simulink model "Likitha_Version_3_1"  (R2025b)
settings: Solver=VariableStepAuto  StartTime=0.0  StopTime=0.3  RelTol=1e-3
undefined symbols (not defined in the file): Ion, Lithium
libraries: spsBatteryLib x50, spsSeriesRLCBranchLib x15, spsCurrentMeasurementLib x10, spsVoltageMeasurementLib x10, spsIdealSwitchLib x9, spsMosfetLib x7, slpidlib x4, spsPWMGeneratorDCDCLib x2, spspowerguiLib x2, spsACVoltageSourceLib x1, eeHysteresisControl x1, spsDCMachineLib x1
(part 2 of 3)

== system Likitha_Version_3_1/Subsystem/Pulse Generator ==
  N,ref : Inport
  N,actual : Inport  Port=2
  Discrete PID Controller : slpidlib/PID Controller  Controller=PI  Form=Parallel  TimeDomain=Discrete-time  UseExternalTs=off  SampleTime=-1  IntegratorMethod=Forward Euler  FilterMethod=Forward Euler  ControllerParametersSource=internal  P=0.002  I=3e-3  UseKiTs=off  D=0  UseExternalDerivativeSource=off  N=100  UseFilter=on  TunerSelectOption=Transfer Function Based (PID Tuner App)  InitialConditionSource=internal  InitialConditionForIntegrator=0  InitialConditionForFilter=0  DifferentiatorICPrevScaledInput=0  ExternalReset=none  TrackingMode=off  Kt=1  LimitOutput=off  SatLimitsSource=internal  UpperSaturationLimit=inf  LowerSaturationLimit=-inf  LinearizeAsGain=off  AntiWindupMode=none  Kb=1  LimitIntegrator=off  UpperIntegratorSaturationLimit=inf  LowerIntegratorSaturationLimit=-inf  POutMin=[]  POutMax=[]  IOutMin=[]  IOutMax=[]  DOutMin=[]  DOutMax=[]  NOutMin=[]  NOutMax=[]  SumOutMin=[]  SumOutMax=[]  SaturationOutMin=[]  SaturationOutMax=[]  PParamMin=[]  PParamMax=[]  IParamMin=[]  IParamMax=[]  DParamMin=[]  DParamMax=[]  NParamMin=[]  NParamMax=[]  KbParamMin=[]  KbParamMax=[]  KtParamMin=[]  KtParamMax=[]  KbOutMin=[]  KbOutMax=[]  KtOutMin=[]  KtOutMax=[]  IntegratorOutMin=[]  IntegratorOutMax=[]  FilterOutMin=[]  FilterOutMax=[]  SumI1OutMin=[]  SumI1OutMax=[]  SumI2OutMin=[]  SumI2OutMax=[]  SumI3OutMin=[]  SumI3OutMax=[]  SumI4OutMin=[]  SumI4OutMax=[]  SumDOutMin=[]  SumDOutMax=[]  DifferentiatorOutMin=[]  DifferentiatorOutMax=[]  FilterDiffOutCoefMin=[]  FilterDiffOutCoefMax=[]  ReciprocalOutMin=[]  ReciprocalOutMax=[]  SumDenOutMin=[]  SumDenOutMax=[]  SumNumOutMin=[]  SumNumOutMax=[]  DivideOutMin=[]  DivideOutMax=[]  UdiffTsProdOutMin=[]  UdiffTsProdOutMax=[]  NTsProdOutMin=[]  NTsProdOutMax=[]  UintegralTsProdOutMin=[]  UintegralTsProdOutMax=[]  UngainTsProdOutMin=[]  UngainTsProdOutMax=[]  ClampingZeroOutDataTypeStr=Inherit: Inherit via back propagation  ClampingZeroOutMin=[]  ClampingZeroOutMax=[]  FilterDenConstantOutDataTypeStr=Inherit: Inherit via back propagation  FilterDenConstantOutMin=[]  FilterDenConstantOutMax=[]  PCopyOutDataTypeStr=Inherit: Inherit via back propagation  PCopyOutMin=[]  PCopyOutMax=[]  NCopyOutDataTypeStr=Inherit: Inherit via back propagation  NCopyOutMin=[]  NCopyOutMax=[]  IntegratorContinuousStateAttributes=''  IntegratorStateMustResolveToSignalObject=off  IntegratorRTWStateStorageClass=Auto  FilterContinuousStateAttributes=''  FilterStateMustResolveToSignalObject=off  FilterRTWStateStorageClass=Auto  ParallelPVariant=InternalParameters  IdealPVariant=Disabled  IVariant=InternalParameters  DVariant=Disabled  IntegratorVariant=Discrete  SatVariant=Disabled  AWVariant=Passthrough  PCopyVariant=Disabled  TRVariant=Disabled  FdbkBlocksVariant=Forward  IdealPFdbkVariant=Disabled  SatFdbkVariant=Disabled  DerivativeFilterVariant=Disabled  NVariant=Disabled  NCopyVariant=Disabled_SignalSpec  FilterICVariant=Disabled  IntegratorICVariant=InternalICs  ExternalResetVariant=Disabled  TRSumVariant=Passthrough  SumFdbkVariant=Disabled  SumVariant=Sum_PI  TsampFilterVariant=InternalTs  TsampNgainVariant=Passthrough  TsampIntegralVariant=Disabled_SignalSpec  ExternalSaturationOutDataTypeStr=Inherit: Same as second input  DerivativeSourceVariant=Disabled  PreIntVariant=InternalPreInt
  Gain : Gain  Gain=0.9
  Relational Operator : RelationalOperator  OutDataTypeStr=boolean  RndMeth=Simplest  InputSameDT=off
  Saturation : Saturate  UpperLimit=1  LowerLimit=-1
  Sawtooth Generator : spsSawtoothGeneratorLib/Sawtooth Generator  Freq=2e3  Phase=0  Ts=0
  Subtract : Sum  Inputs=+-
  pulse : Outport
  wires:
  Gain/1 -> Relational Operator/1
  Subtract/1 -> Discrete PID Controller/1
  Sawtooth Generator/1 -> Relational Operator/2
  Discrete PID Controller/1 -> Saturation/1
  Saturation/1 -> Gain/1
  Relational Operator/1 -> pulse/1
  N,actual/1 -> Subtract/2
  N,ref/1 -> Subtract/1

== system Likitha_Version_3_1/Subsystem11/1 ==
  Battery1 : spsBatteryLib/Battery  BatType=Lithium-Ion  NomV=3.3  NomQ=2.5  SOC=60  Batt_Tr=30  PresetModel=off  MaxQ=2.5  MinV=2.475  FullV=3.8412  Dis_rate=1.1739  R=0.05  Normal_OP=2.4417  expZone="[3.5653     0.13265]"
  Bus Selector : BusSelector  OutputSignals=SOC (%),Current (A),Voltage (V)
  Product : Product
  Scope : Scope  NumInputPorts=4
      settings: ActiveDisplayYMinimum=50.396039603960396  ActiveDisplayYMaximum=70.396039603960389
  Series RLC Branch : spsSeriesRLCBranchLib/Series RLC Branch  LConnTagsString=__new0  RConnTagsString=__new0  BranchType=R  Resistance=10  Inductance=1e-3  SetiL0=off  InitialCurrent=0  Capacitance=1e-6  Setx0=off  InitialVoltage=0  Measurements=None
  powergui : spspowerguiLib/powergui  Priority=1  SimulationMode=Continuous  SampleTime=50e-6  frequency=60  Iterations=50  frequencyindice=60  Pbase=100e6  ErrMax=1e-4  UnitsV=kV  UnitsW=MW  buscounter=0  FunctionMessages=off  echomessages=off  EnableUseOfTLC=off  CurrentSourceSwitches=off  DisableSnubberDevices=off  DisableRonSwitches=off  DisableVfSwitches=off  DisplayEquations=off  AutomaticDiscreteSolvers=off  SolverType=Tustin/Backward Euler (TBE)  Interpol=off  ExternalGateDelay=off  methode=off  Ts=100  x0status=blocks  SPID=on  SwTol=0  HookPort=off  NonlinearTolerance=1e-4  nMaxIteration=100  ContinueOnMaxIteration=off  RestoreLinks=warning  ResistiveCurrentMeasurement=off  Frange=[0:2:500]  Ylog=off  Xlog=on  ShowGrid=off  save=off  variable=ZData  structure=0  ZoomFFT=off  StartTime=0.0  cycles=1  DisplayStyle=1  fundamental=60  FreqAxis=off  MaxFrequency=1000  frequencyindicesteady=1  RmsSteady=1  display=off
  + : PMIOPort  Side=Right
  - : PMIOPort  Port=2  Side=Right
  tag scope: cm_1=global, soc1=global, vm_1=global
  wires:
  Battery1/1 -> Bus Selector/1
  Bus Selector/3 -> [vm_1], Scope/3, Product/2  "<Voltage (V)>"
  Bus Selector/1 -> [soc1], Scope/1  "<SOC (%)>"
  Bus Selector/2 -> [cm_1], Scope/2, Product/1  "<Current (A)>"
  Product/1 -> Scope/4
  connections:
  -/RConn1 -- Battery1/LConn2 -- Series RLC Branch/RConn1
  +/RConn1 -- Battery1/LConn1 -- Series RLC Branch/LConn1

== system Likitha_Version_3_1/Subsystem11/10 ==
  Battery1 : spsBatteryLib/Battery  BatType=Lithium-Ion  NomV=3.3  NomQ=2.7  SOC=95.5  Batt_Tr=30  PresetModel=on  MaxQ=2.7  MinV=2.475  FullV=3.8412  Dis_rate=1.1739  R=0.012222  Normal_OP=2.4417  expZone="[3.5653     0.13265]"
  Bus Selector : BusSelector  OutputSignals=SOC (%),Current (A),Voltage (V)
  Product : Product
  Scope : Scope  NumInputPorts=4
      settings: ActiveDisplayYMinimum=99.92989  ActiveDisplayYMaximum=100.00779
  + : PMIOPort  Side=Right
  - : PMIOPort  Port=2  Side=Right
  tag scope: cm_10=global, soc10=global, vm_10=global
  wires:
  Battery1/1 -> Bus Selector/1
  Bus Selector/1 -> [soc10], Scope/1  "<SOC (%)>"
  Product/1 -> Scope/4
  Bus Selector/2 -> [cm_10], Product/1, Scope/2  "<Current (A)>"
  Bus Selector/3 -> [vm_10], Scope/3, Product/2  "<Voltage (V)>"
  connections:
  +/RConn1 -- Battery1/LConn1
  -/RConn1 -- Battery1/LConn2

== system Likitha_Version_3_1/Subsystem11/11 ==
  Battery1 : spsBatteryLib/Battery  BatType=Lithium-Ion  NomV=3.3  NomQ=2.7  SOC=90  Batt_Tr=30  PresetModel=on  MaxQ=2.7  MinV=2.475  FullV=3.8412  Dis_rate=1.1739  R=0.012222  Normal_OP=2.4417  expZone="[3.5653     0.13265]"
  Bus Selector : BusSelector  OutputSignals=SOC (%),Current (A),Voltage (V)
  Product : Product
  Scope : Scope  NumInputPorts=4
      settings: ActiveDisplayYMinimum=99.92989  ActiveDisplayYMaximum=100.00779
  Series RLC Branch : spsSeriesRLCBranchLib/Series RLC Branch  LConnTagsString=__new0  RConnTagsString=__new0  BranchType=R  Resistance=0.01  Inductance=1e-3  SetiL0=off  InitialCurrent=0  Capacitance=1e-6  Setx0=off  InitialVoltage=0  Measurements=None
  + : PMIOPort  Side=Right
  - : PMIOPort  Port=2  Side=Right
  tag scope: cm_11=global, soc11=global, vm_11=global
  wires:
  Battery1/1 -> Bus Selector/1
  Bus Selector/1 -> [soc11], Scope/1  "<SOC (%)>"
  Product/1 -> Scope/4
  Bus Selector/2 -> [cm_11], Product/1, Scope/2  "<Current (A)>"
  Bus Selector/3 -> [vm_11], Scope/3, Product/2  "<Voltage (V)>"
  connections:
  -/RConn1 -- Battery1/LConn2
  Series RLC Branch/LConn1 -- Battery1/LConn1
  Series RLC Branch/RConn1 -- +/RConn1

== system Likitha_Version_3_1/Subsystem11/12 ==
  Battery1 : spsBatteryLib/Battery  BatType=Lithium-Ion  NomV=3.264  NomQ=2.61  SOC=81  Batt_Tr=30  PresetModel=on  MaxQ=2.61  MinV=2.448  FullV=3.7993  Dis_rate=1.1348  R=0.012506  Normal_OP=2.3603  expZone="[3.5264     0.12823]"
  Bus Selector : BusSelector  OutputSignals=SOC (%),Current (A),Voltage (V)
  Product : Product
  Scope : Scope  NumInputPorts=4
      settings: ActiveDisplayYMinimum=99.92989  ActiveDisplayYMaximum=100.00779
  + : PMIOPort  Side=Right
  - : PMIOPort  Port=2  Side=Right
  tag scope: cm_20=global, soc20=global, vm_20=global
  wires:
  Battery1/1 -> Bus Selector/1
  Bus Selector/1 -> [soc20], Scope/1  "<SOC (%)>"
  Product/1 -> Scope/4
  Bus Selector/2 -> [cm_20], Product/1, Scope/2  "<Current (A)>"
  Bus Selector/3 -> [vm_20], Scope/3, Product/2  "<Voltage (V)>"
  connections:
  +/RConn1 -- Battery1/LConn1
  -/RConn1 -- Battery1/LConn2

== system Likitha_Version_3_1/Subsystem11/13 ==
  Battery1 : spsBatteryLib/Battery  BatType=Lithium-Ion  NomV=3.296  NomQ=2.69  SOC=89  Batt_Tr=30  PresetModel=on  MaxQ=2.69  MinV=2.472  FullV=3.8365  Dis_rate=1.1696  R=0.012253  Normal_OP=2.4327  expZone="[3.561     0.13216]"
  Bus Selector : BusSelector  OutputSignals=SOC (%),Current (A),Voltage (V)
  Product : Product
  Scope : Scope  NumInputPorts=4
      settings: ActiveDisplayYMinimum=99.92989  ActiveDisplayYMaximum=100.00779
  + : PMIOPort  Side=Right
  - : PMIOPort  Port=2  Side=Right
  tag scope: cm_12=global, soc12=global, vm_12=global
  wires:
  Battery1/1 -> Bus Selector/1
  Bus Selector/1 -> [soc12], Scope/1  "<SOC (%)>"
  Product/1 -> Scope/4
  Bus Selector/2 -> [cm_12], Product/1, Scope/2  "<Current (A)>"
  Bus Selector/3 -> [vm_12], Scope/3, Product/2  "<Voltage (V)>"
  connections:
  +/RConn1 -- Battery1/LConn1
  -/RConn1 -- Battery1/LConn2

== system Likitha_Version_3_1/Subsystem11/14 ==
  Battery1 : spsBatteryLib/Battery  BatType=Lithium-Ion  NomV=3.292  NomQ=2.68  SOC=88  Batt_Tr=30  PresetModel=on  MaxQ=2.68  MinV=2.469  FullV=3.8318  Dis_rate=1.1652  R=0.012284  Normal_OP=2.4237  expZone="[3.5566     0.13167]"
  Bus Selector : BusSelector  OutputSignals=SOC (%),Current (A),Voltage (V)
  Product : Product
  Scope : Scope  NumInputPorts=4
      settings: ActiveDisplayYMinimum=99.92989  ActiveDisplayYMaximum=100.00779
  + : PMIOPort  Side=Right
  - : PMIOPort  Port=2  Side=Right
  tag scope: cm_13=global, soc13=global, vm_13=global
  wires:
  Battery1/1 -> Bus Selector/1
  Bus Selector/1 -> [soc13], Scope/1  "<SOC (%)>"
  Product/1 -> Scope/4
  Bus Selector/2 -> [cm_13], Product/1, Scope/2  "<Current (A)>"
  Bus Selector/3 -> [vm_13], Scope/3, Product/2  "<Voltage (V)>"
  connections:
  +/RConn1 -- Battery1/LConn1
  -/RConn1 -- Battery1/LConn2

== system Likitha_Version_3_1/Subsystem11/15 ==
  Battery1 : spsBatteryLib/Battery  BatType=Lithium-Ion  NomV=3.288  NomQ=2.67  SOC=87  Batt_Tr=30  PresetModel=on  MaxQ=2.67  MinV=2.466  FullV=3.8272  Dis_rate=1.1609  R=0.012315  Normal_OP=2.4146  expZone="[3.5523     0.13118]"
  Bus Selector : BusSelector  OutputSignals=SOC (%),Current (A),Voltage (V)
  Product : Product
  Scope : Scope  NumInputPorts=4
      settings: ActiveDisplayYMinimum=99.92989  ActiveDisplayYMaximum=100.00779
  + : PMIOPort  Side=Right
  - : PMIOPort  Port=2  Side=Right
  tag scope: cm_14=global, soc14=global, vm_14=global
  wires:
  Battery1/1 -> Bus Selector/1
  Bus Selector/1 -> [soc14], Scope/1  "<SOC (%)>"
  Product/1 -> Scope/4
  Bus Selector/2 -> [cm_14], Product/1, Scope/2  "<Current (A)>"
  Bus Selector/3 -> [vm_14], Scope/3, Product/2  "<Voltage (V)>"
  connections:
  +/RConn1 -- Battery1/LConn1
  -/RConn1 -- Battery1/LConn2

== system Likitha_Version_3_1/Subsystem11/16 ==
  Battery1 : spsBatteryLib/Battery  BatType=Lithium-Ion  NomV=3.284  NomQ=2.66  SOC=86  Batt_Tr=30  PresetModel=on  MaxQ=2.66  MinV=2.463  FullV=3.8225  Dis_rate=1.1565  R=0.012346  Normal_OP=2.4056  expZone="[3.548     0.13069]"
  Bus Selector : BusSelector  OutputSignals=SOC (%),Current (A),Voltage (V)
  Product : Product
  Scope : Scope  NumInputPorts=4
      settings: ActiveDisplayYMinimum=99.92989  ActiveDisplayYMaximum=100.00779
  + : PMIOPort  Side=Right
  - : PMIOPort  Port=2  Side=Right
  tag scope: cm_15=global, soc15=global, vm_15=global
  wires:
  Battery1/1 -> Bus Selector/1
  Bus Selector/1 -> [soc15], Scope/1  "<SOC (%)>"
  Product/1 -> Scope/4
  Bus Selector/2 -> [cm_15], Product/1, Scope/2  "<Current (A)>"
  Bus Selector/3 -> [vm_15], Scope/3, Product/2  "<Voltage (V)>"
  connections:
  +/RConn1 -- Battery1/LConn1
  -/RConn1 -- Battery1/LConn2

== system Likitha_Version_3_1/Subsystem11/17 ==
  Battery1 : spsBatteryLib/Battery  BatType=Lithium-Ion  NomV=3.28  NomQ=2.65  SOC=85  Batt_Tr=30  PresetModel=on  MaxQ=2.65  MinV=2.46  FullV=3.8179  Dis_rate=1.1522  R=0.012377  Normal_OP=2.3965  expZone="[3.5437      0.1302]"
  Bus Selector : BusSelector  OutputSignals=SOC (%),Current (A),Voltage (V)
  Product : Product
  Scope : Scope  NumInputPorts=4
      settings: ActiveDisplayYMinimum=99.92989  ActiveDisplayYMaximum=100.00779
  + : PMIOPort  Side=Right
  - : PMIOPort  Port=2  Side=Right
  tag scope: cm_16=global, soc16=global, vm_16=global
  wires:
  Battery1/1 -> Bus Selector/1
  Bus Selector/1 -> [soc16], Scope/1  "<SOC (%)>"
  Product/1 -> Scope/4
  Bus Selector/2 -> [cm_16], Product/1, Scope/2  "<Current (A)>"
  Bus Selector/3 -> [vm_16], Scope/3, Product/2  "<Voltage (V)>"
  connections:
  +/RConn1 -- Battery1/LConn1
  -/RConn1 -- Battery1/LConn2

== system Likitha_Version_3_1/Subsystem11/18 ==
  Battery1 : spsBatteryLib/Battery  BatType=Lithium-Ion  NomV=3.276  NomQ=2.64  SOC=84  Batt_Tr=30  PresetModel=on  MaxQ=2.64  MinV=2.457  FullV=3.8132  Dis_rate=1.1478  R=0.012409  Normal_OP=2.3875  expZone="[3.5393      0.1297]"
  Bus Selector : BusSelector  OutputSignals=SOC (%),Current (A),Voltage (V)
  Product : Product
  Scope : Scope  NumInputPorts=4
      settings: ActiveDisplayYMinimum=99.92989  ActiveDisplayYMaximum=100.00779
  + : PMIOPort  Side=Right
  - : PMIOPort  Port=2  Side=Right
  tag scope: cm_17=global, soc17=global, vm_17=global
  wires:
  Battery1/1 -> Bus Selector/1
  Bus Selector/1 -> [soc17], Scope/1  "<SOC (%)>"
  Product/1 -> Scope/4
  Bus Selector/2 -> [cm_17], Product/1, Scope/2  "<Current (A)>"
  Bus Selector/3 -> [vm_17], Scope/3, Product/2  "<Voltage (V)>"
  connections:
  +/RConn1 -- Battery1/LConn1
  -/RConn1 -- Battery1/LConn2

== system Likitha_Version_3_1/Subsystem11/19 ==
  Battery1 : spsBatteryLib/Battery  BatType=Lithium-Ion  NomV=3.272  NomQ=2.63  SOC=83  Batt_Tr=30  PresetModel=on  MaxQ=2.63  MinV=2.454  FullV=3.8086  Dis_rate=1.1435  R=0.012441  Normal_OP=2.3784  expZone="[3.535     0.12921]"
  Bus Selector : BusSelector  OutputSignals=SOC (%),Current (A),Voltage (V)
  Product : Product
  Scope : Scope  NumInputPorts=4
      settings: ActiveDisplayYMinimum=99.92989  ActiveDisplayYMaximum=100.00779
  + : PMIOPort  Side=Right
  - : PMIOPort  Port=2  Side=Right
  tag scope: cm_18=global, soc18=global, vm_18=global
  wires:
  Battery1/1 -> Bus Selector/1
  Bus Selector/1 -> [soc18], Scope/1  "<SOC (%)>"
  Product/1 -> Scope/4
  Bus Selector/2 -> [cm_18], Product/1, Scope/2  "<Current (A)>"
  Bus Selector/3 -> [vm_18], Scope/3, Product/2  "<Voltage (V)>"
  connections:
  +/RConn1 -- Battery1/LConn1
  -/RConn1 -- Battery1/LConn2

== system Likitha_Version_3_1/Subsystem11/2 ==
  Battery1 : spsBatteryLib/Battery  BatType=Lithium-Ion  NomV=3.3  NomQ=2.7  SOC=99.5  Batt_Tr=30  PresetModel=on  MaxQ=2.7  MinV=2.475  FullV=3.8412  Dis_rate=1.1739  R=0.012222  Normal_OP=2.4417  expZone="[3.5653     0.13265]"
  Bus Selector : BusSelector  OutputSignals=SOC (%),Current (A),Voltage (V)
  Product : Product
  Scope : Scope  NumInputPorts=4
      settings: ActiveDisplayYMinimum=99.92989  ActiveDisplayYMaximum=100.00779
  + : PMIOPort  Side=Right
  - : PMIOPort  Port=2  Side=Right
  tag scope: cm_2=global, soc2=global, vm_2=global
  wires:
  Battery1/1 -> Bus Selector/1
  Bus Selector/1 -> [soc2], Scope/1  "<SOC (%)>"
  Product/1 -> Scope/4
  Bus Selector/2 -> Product/1, [cm_2], Scope/2  "<Current (A)>"
  Bus Selector/3 -> [vm_2], Scope/3, Product/2  "<Voltage (V)>"
  connections:
  +/RConn1 -- Battery1/LConn1
  -/RConn1 -- Battery1/LConn2

== system Likitha_Version_3_1/Subsystem11/20 ==
  Battery1 : spsBatteryLib/Battery  BatType=Lithium-Ion  NomV=3.268  NomQ=2.62  SOC=82  Batt_Tr=30  PresetModel=on  MaxQ=2.62  MinV=2.451  FullV=3.8039  Dis_rate=1.1391  R=0.012473  Normal_OP=2.3694  expZone="[3.5307     0.12872]"
  Bus Selector : BusSelector  OutputSignals=SOC (%),Current (A),Voltage (V)
  Product : Product
  Scope : Scope  NumInputPorts=4
      settings: ActiveDisplayYMinimum=99.92989  ActiveDisplayYMaximum=100.00779
  + : PMIOPort  Side=Right
  - : PMIOPort  Port=2  Side=Right
  tag scope: cm_19=global, soc19=global, vm_19=global
  wires:
  Battery1/1 -> Bus Selector/1
  Bus Selector/1 -> [soc19], Scope/1  "<SOC (%)>"
  Product/1 -> Scope/4
  Bus Selector/2 -> [cm_19], Product/1, Scope/2  "<Current (A)>"
  Bus Selector/3 -> [vm_19], Scope/3, Product/2  "<Voltage (V)>"
  connections:
  +/RConn1 -- Battery1/LConn1
  -/RConn1 -- Battery1/LConn2

== system Likitha_Version_3_1/Subsystem11/21 ==
  Battery1 : spsBatteryLib/Battery  BatType=Lithium-Ion  NomV=3.25  NomQ=2.6  SOC=80  Batt_Tr=30  PresetModel=on  MaxQ=2.6  MinV=2.4375  FullV=3.783  Dis_rate=1.1304  R=0.0125  Normal_OP=2.3513  expZone="[3.5113     0.12774]"
  Bus Selector : BusSelector  OutputSignals=SOC (%),Current (A),Voltage (V)
  Product : Product
  Scope : Scope  NumInputPorts=4
      settings: ActiveDisplayYMinimum=99.92989  ActiveDisplayYMaximum=100.00779
  Series RLC Branch : spsSeriesRLCBranchLib/Series RLC Branch  LConnTagsString=__new0  RConnTagsString=__new0  BranchType=R  Resistance=0.01  Inductance=1e-3  SetiL0=off  InitialCurrent=0  Capacitance=1e-6  Setx0=off  InitialVoltage=0  Measurements=None
  + : PMIOPort  Side=Right
  - : PMIOPort  Port=2  Side=Right
  tag scope: cm_21=global, soc21=global, vm_21=global
  wires:
  Battery1/1 -> Bus Selector/1
  Bus Selector/1 -> [soc21], Scope/1  "<SOC (%)>"
  Product/1 -> Scope/4
  Bus Selector/2 -> [cm_21], Product/1, Scope/2  "<Current (A)>"
  Bus Selector/3 -> [vm_21], Scope/3, Product/2  "<Voltage (V)>"
  connections:
  -/RConn1 -- Battery1/LConn2
  Series RLC Branch/LConn1 -- Battery1/LConn1
  Series RLC Branch/RConn1 -- +/RConn1

== system Likitha_Version_3_1/Subsystem11/22 ==
  Battery1 : spsBatteryLib/Battery  BatType=Lithium-Ion  NomV=3.205  NomQ=2.51  SOC=71  Batt_Tr=30  PresetModel=on  MaxQ=2.51  MinV=2.4038  FullV=3.7306  Dis_rate=1.0913  R=0.012769  Normal_OP=2.2699  expZone="[3.4626     0.12332]"
  Bus Selector : BusSelector  OutputSignals=SOC (%),Current (A),Voltage (V)
  Product : Product
  Scope : Scope  NumInputPorts=4
      settings: ActiveDisplayYMinimum=99.92989  ActiveDisplayYMaximum=100.00779
  + : PMIOPort  Side=Right
  - : PMIOPort  Port=2  Side=Right
  tag scope: cm_30=global, soc30=global, vm_30=global
  wires:
  Battery1/1 -> Bus Selector/1
  Bus Selector/1 -> [soc30], Scope/1  "<SOC (%)>"
  Product/1 -> Scope/4
  Bus Selector/2 -> [cm_30], Product/1, Scope/2  "<Current (A)>"
  Bus Selector/3 -> [vm_30], Scope/3, Product/2  "<Voltage (V)>"
  connections:
  +/RConn1 -- Battery1/LConn1
  -/RConn1 -- Battery1/LConn2

== system Likitha_Version_3_1/Subsystem11/23 ==
  Battery1 : spsBatteryLib/Battery  BatType=Lithium-Ion  NomV=3.2  NomQ=2.5  SOC=70  Batt_Tr=30  PresetModel=on  MaxQ=2.5  MinV=2.4  FullV=3.7248  Dis_rate=1.087  R=0.0128  Normal_OP=2.2609  expZone="[3.4572     0.12283]"
  Bus Selector : BusSelector  OutputSignals=SOC (%),Current (A),Voltage (V)
  Product : Product
  Scope : Scope  NumInputPorts=4
      settings: ActiveDisplayYMinimum=99.92989  ActiveDisplayYMaximum=100.00779
  Series RLC Branch : spsSeriesRLCBranchLib/Series RLC Branch  LConnTagsString=__new0  RConnTagsString=__new0  BranchType=R  Resistance=0.01  Inductance=1e-3  SetiL0=off  InitialCurrent=0  Capacitance=1e-6  Setx0=off  InitialVoltage=0  Measurements=None
  + : PMIOPort  Side=Right
  - : PMIOPort  Port=2  Side=Right
  tag scope: cm_31=global, soc31=global, vm_31=global
  wires:
  Battery1/1 -> Bus Selector/1
  Bus Selector/1 -> [soc31], Scope/1  "<SOC (%)>"
  Product/1 -> Scope/4
  Bus Selector/2 -> [cm_31], Product/1, Scope/2  "<Current (A)>"
  Bus Selector/3 -> [vm_31], Scope/3, Product/2  "<Voltage (V)>"
  connections:
  -/RConn1 -- Battery1/LConn2
  Series RLC Branch/LConn1 -- Battery1/LConn1
  Series RLC Branch/RConn1 -- +/RConn1

== system Likitha_Version_3_1/Subsystem11/24 ==
  Battery1 : spsBatteryLib/Battery  BatType=Lithium-Ion  NomV=3.155  NomQ=2.41  SOC=61  Batt_Tr=30  PresetModel=on  MaxQ=2.41  MinV=2.3662  FullV=3.6724  Dis_rate=1.0478  R=0.013091  Normal_OP=2.1795  expZone="[3.4086      0.1184]"
  Bus Selector : BusSelector  OutputSignals=SOC (%),Current (A),Voltage (V)
  Product : Product
  Scope : Scope  NumInputPorts=4
      settings: ActiveDisplayYMinimum=99.92989  ActiveDisplayYMaximum=100.00779
  + : PMIOPort  Side=Right
  - : PMIOPort  Port=2  Side=Right
  tag scope: cm_40=global, soc40=global, vm_40=global
  wires:
  Battery1/1 -> Bus Selector/1
  Bus Selector/1 -> [soc40], Scope/1  "<SOC (%)>"
  Product/1 -> Scope/4
  Bus Selector/2 -> [cm_40], Product/1, Scope/2  "<Current (A)>"
  Bus Selector/3 -> [vm_40], Scope/3, Product/2  "<Voltage (V)>"
  connections:
  +/RConn1 -- Battery1/LConn1
  -/RConn1 -- Battery1/LConn2

== system Likitha_Version_3_1/Subsystem11/25 ==
  Battery1 : spsBatteryLib/Battery  BatType=Lithium-Ion  NomV=3.195  NomQ=2.49  SOC=69  Batt_Tr=30  PresetModel=on  MaxQ=2.49  MinV=2.3962  FullV=3.7189  Dis_rate=1.0826  R=0.012831  Normal_OP=2.2518  expZone="[3.4518     0.12233]"
  Bus Selector : BusSelector  OutputSignals=SOC (%),Current (A),Voltage (V)
  Product : Product
  Scope : Scope  NumInputPorts=4
      settings: ActiveDisplayYMinimum=99.92989  ActiveDisplayYMaximum=100.00779
  + : PMIOPort  Side=Right
  - : PMIOPort  Port=2  Side=Right
  tag scope: cm_32=global, soc32=global, vm_32=global
  wires:
  Battery1/1 -> Bus Selector/1
  Bus Selector/1 -> [soc32], Scope/1  "<SOC (%)>"
  Product/1 -> Scope/4
  Bus Selector/2 -> [cm_32], Product/1, Scope/2  "<Current (A)>"
  Bus Selector/3 -> [vm_32], Scope/3, Product/2  "<Voltage (V)>"
  connections:
  +/RConn1 -- Battery1/LConn1
  -/RConn1 -- Battery1/LConn2

== system Likitha_Version_3_1/Subsystem11/26 ==
  Battery1 : spsBatteryLib/Battery  BatType=Lithium-Ion  NomV=3.19  NomQ=2.48  SOC=68  Batt_Tr=30  PresetModel=on  MaxQ=2.48  MinV=2.3925  FullV=3.7131  Dis_rate=1.0783  R=0.012863  Normal_OP=2.2428  expZone="[3.4464     0.12184]"
  Bus Selector : BusSelector  OutputSignals=SOC (%),Current (A),Voltage (V)
  Product : Product
  Scope : Scope  NumInputPorts=4
      settings: ActiveDisplayYMinimum=99.92989  ActiveDisplayYMaximum=100.00779
  + : PMIOPort  Side=Right
  - : PMIOPort  Port=2  Side=Right
  tag scope: cm_33=global, soc33=global, vm_33=global
  wires:
  Battery1/1 -> Bus Selector/1
  Bus Selector/1 -> [soc33], Scope/1  "<SOC (%)>"
  Product/1 -> Scope/4
  Bus Selector/2 -> [cm_33], Product/1, Scope/2  "<Current (A)>"
  Bus Selector/3 -> [vm_33], Scope/3, Product/2  "<Voltage (V)>"
  connections:
  +/RConn1 -- Battery1/LConn1
  -/RConn1 -- Battery1/LConn2

== system Likitha_Version_3_1/Subsystem11/27 ==
  Battery1 : spsBatteryLib/Battery  BatType=Lithium-Ion  NomV=3.185  NomQ=2.47  SOC=67  Batt_Tr=30  PresetModel=on  MaxQ=2.47  MinV=2.3887  FullV=3.7073  Dis_rate=1.0739  R=0.012895  Normal_OP=2.2337  expZone="[3.441     0.12135]"
  Bus Selector : BusSelector  OutputSignals=SOC (%),Current (A),Voltage (V)
  Product : Product
  Scope : Scope  NumInputPorts=4
      settings: ActiveDisplayYMinimum=99.92989  ActiveDisplayYMaximum=100.00779
  + : PMIOPort  Side=Right
  - : PMIOPort  Port=2  Side=Right
  tag scope: cm_34=global, soc34=global, vm_34=global
  wires:
  Battery1/1 -> Bus Selector/1
  Bus Selector/1 -> [soc34], Scope/1  "<SOC (%)>"
  Product/1 -> Scope/4
  Bus Selector/2 -> [cm_34], Product/1, Scope/2  "<Current (A)>"
  Bus Selector/3 -> [vm_34], Scope/3, Product/2  "<Voltage (V)>"
  connections:
  +/RConn1 -- Battery1/LConn1
  -/RConn1 -- Battery1/LConn2

== system Likitha_Version_3_1/Subsystem11/28 ==
  Battery1 : spsBatteryLib/Battery  BatType=Lithium-Ion  NomV=3.18  NomQ=2.46  SOC=66  Batt_Tr=30  PresetModel=on  MaxQ=2.46  MinV=2.385  FullV=3.7015  Dis_rate=1.0696  R=0.012927  Normal_OP=2.2247  expZone="[3.4356     0.12086]"
  Bus Selector : BusSelector  OutputSignals=SOC (%),Current (A),Voltage (V)
  Product : Product
  Scope : Scope  NumInputPorts=4
      settings: ActiveDisplayYMinimum=99.92989  ActiveDisplayYMaximum=100.00779
  + : PMIOPort  Side=Right
  - : PMIOPort  Port=2  Side=Right
  tag scope: cm_35=global, soc35=global, vm_35=global
  wires:
  Battery1/1 -> Bus Selector/1
  Bus Selector/1 -> [soc35], Scope/1  "<SOC (%)>"
  Product/1 -> Scope/4
  Bus Selector/2 -> [cm_35], Product/1, Scope/2  "<Current (A)>"
  Bus Selector/3 -> [vm_35], Scope/3, Product/2  "<Voltage (V)>"
  connections:
  +/RConn1 -- Battery1/LConn1
  -/RConn1 -- Battery1/LConn2

== system Likitha_Version_3_1/Subsystem11/29 ==
  Battery1 : spsBatteryLib/Battery  BatType=Lithium-Ion  NomV=3.175  NomQ=2.45  SOC=65  Batt_Tr=30  PresetModel=on  MaxQ=2.45  MinV=2.3812  FullV=3.6957  Dis_rate=1.0652  R=0.012959  Normal_OP=2.2157  expZone="[3.4302     0.12037]"
  Bus Selector : BusSelector  OutputSignals=SOC (%),Current (A),Voltage (V)
  Product : Product
  Scope : Scope  NumInputPorts=4
      settings: ActiveDisplayYMinimum=99.92989  ActiveDisplayYMaximum=100.00779
  + : PMIOPort  Side=Right
  - : PMIOPort  Port=2  Side=Right
  tag scope: cm_36=global, soc36=global, vm_36=global
  wires:
  Battery1/1 -> Bus Selector/1
  Bus Selector/1 -> [soc36], Scope/1  "<SOC (%)>"
  Product/1 -> Scope/4
  Bus Selector/2 -> [cm_36], Product/1, Scope/2  "<Current (A)>"
  Bus Selector/3 -> [vm_36], Scope/3, Product/2  "<Voltage (V)>"
  connections:
  +/RConn1 -- Battery1/LConn1
  -/RConn1 -- Battery1/LConn2

== system Likitha_Version_3_1/Subsystem11/3 ==
  Battery1 : spsBatteryLib/Battery  BatType=Lithium-Ion  NomV=3.3  NomQ=2.7  SOC=99  Batt_Tr=30  PresetModel=on  MaxQ=2.7  MinV=2.475  FullV=3.8412  Dis_rate=1.1739  R=0.012222  Normal_OP=2.4417  expZone="[3.5653     0.13265]"
  Bus Selector : BusSelector  OutputSignals=SOC (%),Current (A),Voltage (V)
  Product : Product
  Scope : Scope  NumInputPorts=4
      settings: ActiveDisplayYMinimum=99.92989  ActiveDisplayYMaximum=100.00779
  + : PMIOPort  Side=Right
  - : PMIOPort  Port=2  Side=Right
  tag scope: cm_3=global, soc3=global, vm_3=global
  wires:
  Battery1/1 -> Bus Selector/1
  Bus Selector/1 -> [soc3], Scope/1  "<SOC (%)>"
  Product/1 -> Scope/4
  Bus Selector/3 -> [vm_3], Scope/3, Product/2  "<Voltage (V)>"
  Bus Selector/2 -> [cm_3], Product/1, Scope/2  "<Current (A)>"
  connections:
  +/RConn1 -- Battery1/LConn1
  -/RConn1 -- Battery1/LConn2

== system Likitha_Version_3_1/Subsystem11/30 ==
  Battery1 : spsBatteryLib/Battery  BatType=Lithium-Ion  NomV=3.17  NomQ=2.44  SOC=64  Batt_Tr=30  PresetModel=on  MaxQ=2.44  MinV=2.3775  FullV=3.6898  Dis_rate=1.0609  R=0.012992  Normal_OP=2.2066  expZone="[3.4248     0.11988]"
  Bus Selector : BusSelector  OutputSignals=SOC (%),Current (A),Voltage (V)
  Product : Product
  Scope : Scope  NumInputPorts=4
      settings: ActiveDisplayYMinimum=99.92989  ActiveDisplayYMaximum=100.00779
  + : PMIOPort  Side=Right
  - : PMIOPort  Port=2  Side=Right
  tag scope: cm_37=global, soc37=global, vm_37=global
  wires:
  Battery1/1 -> Bus Selector/1
  Bus Selector/1 -> [soc37], Scope/1  "<SOC (%)>"
  Product/1 -> Scope/4
  Bus Selector/2 -> [cm_37], Product/1, Scope/2  "<Current (A)>"
  Bus Selector/3 -> [vm_37], Scope/3, Product/2  "<Voltage (V)>"
  connections:
  +/RConn1 -- Battery1/LConn1
  -/RConn1 -- Battery1/LConn2

== system Likitha_Version_3_1/Subsystem11/31 ==
  Battery1 : spsBatteryLib/Battery  BatType=Lithium-Ion  NomV=3.165  NomQ=2.43  SOC=63  Batt_Tr=30  PresetModel=on  MaxQ=2.43  MinV=2.3738  FullV=3.684  Dis_rate=1.0565  R=0.013025  Normal_OP=2.1976  expZone="[3.4194     0.11939]"
  Bus Selector : BusSelector  OutputSignals=SOC (%),Current (A),Voltage (V)
  Product : Product
  Scope : Scope  NumInputPorts=4
      settings: ActiveDisplayYMinimum=99.92989  ActiveDisplayYMaximum=100.00779
  + : PMIOPort  Side=Right
  - : PMIOPort  Port=2  Side=Right
  tag scope: cm_38=global, soc38=global, vm_38=global
  wires:
  Battery1/1 -> Bus Selector/1
  Bus Selector/1 -> [soc38], Scope/1  "<SOC (%)>"
  Product/1 -> Scope/4
  Bus Selector/2 -> [cm_38], Product/1, Scope/2  "<Current (A)>"
  Bus Selector/3 -> [vm_38], Scope/3, Product/2  "<Voltage (V)>"
  connections:
  +/RConn1 -- Battery1/LConn1
  -/RConn1 -- Battery1/LConn2

== system Likitha_Version_3_1/Subsystem11/32 ==
  Battery1 : spsBatteryLib/Battery  BatType=Lithium-Ion  NomV=3.245  NomQ=2.59  SOC=79  Batt_Tr=30  PresetModel=on  MaxQ=2.59  MinV=2.4337  FullV=3.7771  Dis_rate=1.1261  R=0.012529  Normal_OP=2.3423  expZone="[3.5059     0.12725]"
  Bus Selector : BusSelector  OutputSignals=SOC (%),Current (A),Voltage (V)
  Product : Product
  Scope : Scope  NumInputPorts=4
      settings: ActiveDisplayYMinimum=99.92989  ActiveDisplayYMaximum=100.00779
  + : PMIOPort  Side=Right
  - : PMIOPort  Port=2  Side=Right
  tag scope: cm_22=global, soc22=global, vm_22=global
  wires:
  Battery1/1 -> Bus Selector/1
  Bus Selector/1 -> [soc22], Scope/1  "<SOC (%)>"
  Product/1 -> Scope/4
  Bus Selector/2 -> [cm_22], Product/1, Scope/2  "<Current (A)>"
  Bus Selector/3 -> [vm_22], Scope/3, Product/2  "<Voltage (V)>"
  connections:
  +/RConn1 -- Battery1/LConn1
  -/RConn1 -- Battery1/LConn2

== system Likitha_Version_3_1/Subsystem11/33 ==
  Battery1 : spsBatteryLib/Battery  BatType=Lithium-Ion  NomV=3.16  NomQ=2.42  SOC=62  Batt_Tr=30  PresetModel=on  MaxQ=2.42  MinV=2.37  FullV=3.6782  Dis_rate=1.0522  R=0.013058  Normal_OP=2.1885  expZone="[3.414      0.1189]"
  Bus Selector : BusSelector  OutputSignals=SOC (%),Current (A),Voltage (V)
  Product : Product
  Scope : Scope  NumInputPorts=4
      settings: ActiveDisplayYMinimum=99.92989  ActiveDisplayYMaximum=100.00779
  + : PMIOPort  Side=Right
  - : PMIOPort  Port=2  Side=Right
  tag scope: cm_39=global, soc39=global, vm_39=global
  wires:
  Battery1/1 -> Bus Selector/1
  Bus Selector/1 -> [soc39], Scope/1  "<SOC (%)>"
  Product/1 -> Scope/4
  Bus Selector/2 -> [cm_39], Product/1, Scope/2  "<Current (A)>"
  Bus Selector/3 -> [vm_39], Scope/3, Product/2  "<Voltage (V)>"
  connections:
  +/RConn1 -- Battery1/LConn1
  -/RConn1 -- Battery1/LConn2

== system Likitha_Version_3_1/Subsystem11/34 ==
  Battery1 : spsBatteryLib/Battery  BatType=Lithium-Ion  NomV=3.24  NomQ=2.58  SOC=78  Batt_Tr=30  PresetModel=on  MaxQ=2.58  MinV=2.43  FullV=3.7713  Dis_rate=1.1217  R=0.012558  Normal_OP=2.3332  expZone="[3.5005     0.12676]"
  Bus Selector : BusSelector  OutputSignals=SOC (%),Current (A),Voltage (V)
  Product : Product
  Scope : Scope  NumInputPorts=4
      settings: ActiveDisplayYMinimum=99.92989  ActiveDisplayYMaximum=100.00779
  + : PMIOPort  Side=Right
  - : PMIOPort  Port=2  Side=Right
  tag scope: cm_23=global, soc23=global, vm_23=global
  wires:
  Battery1/1 -> Bus Selector/1
  Bus Selector/1 -> [soc23], Scope/1  "<SOC (%)>"
  Product/1 -> Scope/4
  Bus Selector/2 -> [cm_23], Product/1, Scope/2  "<Current (A)>"
  Bus Selector/3 -> [vm_23], Scope/3, Product/2  "<Voltage (V)>"
  connections:
  +/RConn1 -- Battery1/LConn1
  -/RConn1 -- Battery1/LConn2

== system Likitha_Version_3_1/Subsystem11/35 ==
  Battery1 : spsBatteryLib/Battery  BatType=Lithium-Ion  NomV=3.235  NomQ=2.57  SOC=77  Batt_Tr=30  PresetModel=on  MaxQ=2.57  MinV=2.4263  FullV=3.7655  Dis_rate=1.1174  R=0.012588  Normal_OP=2.3242  expZone="[3.495     0.12627]"
  Bus Selector : BusSelector  OutputSignals=SOC (%),Current (A),Voltage (V)
  Product : Product
  Scope : Scope  NumInputPorts=4
      settings: ActiveDisplayYMinimum=99.92989  ActiveDisplayYMaximum=100.00779
  + : PMIOPort  Side=Right
  - : PMIOPort  Port=2  Side=Right
  tag scope: cm_24=global, soc24=global, vm_24=global
  wires:
  Battery1/1 -> Bus Selector/1
  Bus Selector/1 -> [soc24], Scope/1  "<SOC (%)>"
  Product/1 -> Scope/4
  Bus Selector/2 -> [cm_24], Product/1, Scope/2  "<Current (A)>"
  Bus Selector/3 -> [vm_24], Scope/3, Product/2  "<Voltage (V)>"
  connections:
  +/RConn1 -- Battery1/LConn1
  -/RConn1 -- Battery1/LConn2

== system Likitha_Version_3_1/Subsystem11/36 ==
  Battery1 : spsBatteryLib/Battery  BatType=Lithium-Ion  NomV=3.23  NomQ=2.56  SOC=76  Batt_Tr=30  PresetModel=on  MaxQ=2.56  MinV=2.4225  FullV=3.7597  Dis_rate=1.113  R=0.012617  Normal_OP=2.3151  expZone="[3.4896     0.12577]"
  Bus Selector : BusSelector  OutputSignals=SOC (%),Current (A),Voltage (V)
  Product : Product
  Scope : Scope  NumInputPorts=4
      settings: ActiveDisplayYMinimum=99.92989  ActiveDisplayYMaximum=100.00779
  + : PMIOPort  Side=Right
  - : PMIOPort  Port=2  Side=Right
  tag scope: cm_25=global, soc25=global, vm_25=global
  wires:
  Battery1/1 -> Bus Selector/1
  Bus Selector/1 -> [soc25], Scope/1  "<SOC (%)>"
  Product/1 -> Scope/4
  Bus Selector/2 -> [cm_25], Product/1, Scope/2  "<Current (A)>"
  Bus Selector/3 -> [vm_25], Scope/3, Product/2  "<Voltage (V)>"
  connections:
  +/RConn1 -- Battery1/LConn1
  -/RConn1 -- Battery1/LConn2

== system Likitha_Version_3_1/Subsystem11/37 ==
  Battery1 : spsBatteryLib/Battery  BatType=Lithium-Ion  NomV=3.225  NomQ=2.55  SOC=75  Batt_Tr=30  PresetModel=on  MaxQ=2.55  MinV=2.4188  FullV=3.7539  Dis_rate=1.1087  R=0.012647  Normal_OP=2.3061  expZone="[3.4842     0.12528]"
  Bus Selector : BusSelector  OutputSignals=SOC (%),Current (A),Voltage (V)
  Product : Product
  Scope : Scope  NumInputPorts=4
      settings: ActiveDisplayYMinimum=99.92989  ActiveDisplayYMaximum=100.00779
  + : PMIOPort  Side=Right
  - : PMIOPort  Port=2  Side=Right
  tag scope: cm_26=global, soc26=global, vm_26=global
  wires:
  Battery1/1 -> Bus Selector/1
  Bus Selector/1 -> [soc26], Scope/1  "<SOC (%)>"
  Product/1 -> Scope/4
  Bus Selector/2 -> [cm_26], Product/1, Scope/2  "<Current (A)>"
  Bus Selector/3 -> [vm_26], Scope/3, Product/2  "<Voltage (V)>"
  connections:
  +/RConn1 -- Battery1/LConn1
  -/RConn1 -- Battery1/LConn2

== system Likitha_Version_3_1/Subsystem11/38 ==
  Battery1 : spsBatteryLib/Battery  BatType=Lithium-Ion  NomV=3.22  NomQ=2.54  SOC=74  Batt_Tr=30  PresetModel=on  MaxQ=2.54  MinV=2.415  FullV=3.748  Dis_rate=1.1043  R=0.012677  Normal_OP=2.297  expZone="[3.4788     0.12479]"
  Bus Selector : BusSelector  OutputSignals=SOC (%),Current (A),Voltage (V)
  Product : Product
  Scope : Scope  NumInputPorts=4
      settings: ActiveDisplayYMinimum=99.92989  ActiveDisplayYMaximum=100.00779
  + : PMIOPort  Side=Right
  - : PMIOPort  Port=2  Side=Right
  tag scope: cm_27=global, soc27=global, vm_27=global
  wires:
  Battery1/1 -> Bus Selector/1
  Bus Selector/1 -> [soc27], Scope/1  "<SOC (%)>"
  Product/1 -> Scope/4
  Bus Selector/2 -> [cm_27], Product/1, Scope/2  "<Current (A)>"
  Bus Selector/3 -> [vm_27], Scope/3, Product/2  "<Voltage (V)>"
  connections:
  +/RConn1 -- Battery1/LConn1
  -/RConn1 -- Battery1/LConn2

== system Likitha_Version_3_1/Subsystem11/39 ==
  Battery1 : spsBatteryLib/Battery  BatType=Lithium-Ion  NomV=3.215  NomQ=2.53  SOC=73  Batt_Tr=30  PresetModel=on  MaxQ=2.53  MinV=2.4112  FullV=3.7422  Dis_rate=1.1  R=0.012708  Normal_OP=2.288  expZone="[3.4734      0.1243]"
  Bus Selector : BusSelector  OutputSignals=SOC (%),Current (A),Voltage (V)
  Product : Product
  Scope : Scope  NumInputPorts=4
      settings: ActiveDisplayYMinimum=99.92989  ActiveDisplayYMaximum=100.00779
  + : PMIOPort  Side=Right
  - : PMIOPort  Port=2  Side=Right
  tag scope: cm_28=global, soc28=global, vm_28=global
  wires:
  Battery1/1 -> Bus Selector/1
  Bus Selector/1 -> [soc28], Scope/1  "<SOC (%)>"
  Product/1 -> Scope/4
  Bus Selector/2 -> [cm_28], Product/1, Scope/2  "<Current (A)>"
  Bus Selector/3 -> [vm_28], Scope/3, Product/2  "<Voltage (V)>"
  connections:
  +/RConn1 -- Battery1/LConn1
  -/RConn1 -- Battery1/LConn2

== system Likitha_Version_3_1/Subsystem11/4 ==
  Battery1 : spsBatteryLib/Battery  BatType=Lithium-Ion  NomV=3.3  NomQ=2.7  SOC=98.5  Batt_Tr=30  PresetModel=on  MaxQ=2.7  MinV=2.475  FullV=3.8412  Dis_rate=1.1739  R=0.012222  Normal_OP=2.4417  expZone="[3.5653     0.13265]"
  Bus Selector : BusSelector  OutputSignals=SOC (%),Current (A),Voltage (V)
  Product : Product
  Scope : Scope  NumInputPorts=4
      settings: ActiveDisplayYMinimum=99.92989  ActiveDisplayYMaximum=100.00779
  + : PMIOPort  Side=Right
  - : PMIOPort  Port=2  Side=Right
  tag scope: cm_4=global, soc4=global, vm_4=global
  wires:
  Battery1/1 -> Bus Selector/1
  Bus Selector/1 -> [soc4], Scope/1  "<SOC (%)>"
  Product/1 -> Scope/4
  Bus Selector/2 -> [cm_4], Product/1, Scope/2  "<Current (A)>"
  Bus Selector/3 -> [vm_4], Scope/3, Product/2  "<Voltage (V)>"
  connections:
  +/RConn1 -- Battery1/LConn1
  -/RConn1 -- Battery1/LConn2

== system Likitha_Version_3_1/Subsystem11/40 ==
  Battery1 : spsBatteryLib/Battery  BatType=Lithium-Ion  NomV=3.21  NomQ=2.52  SOC=72  Batt_Tr=30  PresetModel=on  MaxQ=2.52  MinV=2.4075  FullV=3.7364  Dis_rate=1.0957  R=0.012738  Normal_OP=2.279  expZone="[3.468     0.12381]"
  Bus Selector : BusSelector  OutputSignals=SOC (%),Current (A),Voltage (V)
  Product : Product
  Scope : Scope  NumInputPorts=4
      settings: ActiveDisplayYMinimum=99.92989  ActiveDisplayYMaximum=100.00779
  + : PMIOPort  Side=Right
  - : PMIOPort  Port=2  Side=Right
  tag scope: cm_29=global, soc29=global, vm_29=global
  wires:
  Battery1/1 -> Bus Selector/1
  Bus Selector/1 -> [soc29], Scope/1  "<SOC (%)>"
  Product/1 -> Scope/4
  Bus Selector/2 -> [cm_29], Product/1, Scope/2  "<Current (A)>"
  Bus Selector/3 -> [vm_29], Scope/3, Product/2  "<Voltage (V)>"
  connections:
  +/RConn1 -- Battery1/LConn1
  -/RConn1 -- Battery1/LConn2

== system Likitha_Version_3_1/Subsystem11/41 ==
  Battery1 : spsBatteryLib/Battery  BatType=Lithium-Ion  NomV=3.15  NomQ=2.4  SOC=65  Batt_Tr=30  PresetModel=on  MaxQ=2.4  MinV=2.3625  FullV=3.6666  Dis_rate=1.0435  R=0.013125  Normal_OP=2.1704  expZone="[3.4032     0.11791]"
  Bus Selector : BusSelector  OutputSignals=SOC (%),Current (A),Voltage (V)
  Product : Product
  Scope : Scope  NumInputPorts=4
      settings: ActiveDisplayYMinimum=99.92989  ActiveDisplayYMaximum=100.00779
  Series RLC Branch : spsSeriesRLCBranchLib/Series RLC Branch  LConnTagsString=__new0  RConnTagsString=__new0  BranchType=R  Resistance=0.01  Inductance=1e-3  SetiL0=off  InitialCurrent=0  Capacitance=1e-6  Setx0=off  InitialVoltage=0  Measurements=None
  + : PMIOPort  Side=Right
  - : PMIOPort  Port=2  Side=Right
  tag scope: cm_41=global, soc41=global, vm_41=global
  wires:
  Battery1/1 -> Bus Selector/1
  Bus Selector/1 -> [soc41], Scope/1  "<SOC (%)>"
  Product/1 -> Scope/4
  Bus Selector/2 -> [cm_41], Product/1, Scope/2  "<Current (A)>"
  Bus Selector/3 -> [vm_41], Scope/3, Product/2  "<Voltage (V)>"
  connections:
  -/RConn1 -- Battery1/LConn2
  Series RLC Branch/LConn1 -- Battery1/LConn1
  Series RLC Branch/RConn1 -- +/RConn1

== system Likitha_Version_3_1/Subsystem11/42 ==
  Battery1 : spsBatteryLib/Battery  BatType=Lithium-Ion  NomV=3.105  NomQ=2.31  SOC=56  Batt_Tr=30  PresetModel=on  MaxQ=2.31  MinV=2.3287  FullV=3.6142  Dis_rate=1.0043  R=0.013442  Normal_OP=2.089  expZone="[3.3546     0.11349]"
  Bus Selector : BusSelector  OutputSignals=SOC (%),Current (A),Voltage (V)
  Product : Product
  Scope : Scope  NumInputPorts=4
      settings: ActiveDisplayYMinimum=57.404559023926616  ActiveDisplayYMaximum=57.451502898050578
  + : PMIOPort  Side=Right
  - : PMIOPort  Port=2  Side=Right
  tag scope: cm_50=global, soc50=global, vm_50=global
  wires:
  Battery1/1 -> Bus Selector/1
  Bus Selector/1 -> [soc50], Scope/1  "<SOC (%)>"
  Product/1 -> Scope/4
  Bus Selector/2 -> [cm_50], Product/1, Scope/2  "<Current (A)>"
  Bus Selector/3 -> [vm_50], Scope/3, Product/2  "<Voltage (V)>"
  connections:
  +/RConn1 -- Battery1/LConn1
  -/RConn1 -- Battery1/LConn2

== system Likitha_Version_3_1/Subsystem11/43 ==
  Battery1 : spsBatteryLib/Battery  BatType=Lithium-Ion  NomV=3.145  NomQ=2.39  SOC=64  Batt_Tr=30  PresetModel=on  MaxQ=2.39  MinV=2.3588  FullV=3.6607  Dis_rate=1.0391  R=0.013159  Normal_OP=2.1614  expZone="[3.3978     0.11742]"
  Bus Selector : BusSelector  OutputSignals=SOC (%),Current (A),Voltage (V)
  Product : Product
  Scope : Scope  NumInputPorts=4
      settings: ActiveDisplayYMinimum=99.92989  ActiveDisplayYMaximum=100.00779
  + : PMIOPort  Side=Right
  - : PMIOPort  Port=2  Side=Right
  tag scope: cm_42=global, soc42=global, vm_42=global
  wires:
  Battery1/1 -> Bus Selector/1
  Bus Selector/1 -> [soc42], Scope/1  "<SOC (%)>"
  Product/1 -> Scope/4
  Bus Selector/2 -> [cm_42], Product/1, Scope/2  "<Current (A)>"
  Bus Selector/3 -> [vm_42], Scope/3, Product/2  "<Voltage (V)>"
  connections:
  +/RConn1 -- Battery1/LConn1
  -/RConn1 -- Battery1/LConn2

== system Likitha_Version_3_1/Subsystem11/44 ==
  Battery1 : spsBatteryLib/Battery  BatType=Lithium-Ion  NomV=3.14  NomQ=2.38  SOC=63  Batt_Tr=30  PresetModel=on  MaxQ=2.38  MinV=2.355  FullV=3.6549  Dis_rate=1.0348  R=0.013193  Normal_OP=2.1523  expZone="[3.3924     0.11693]"
  Bus Selector : BusSelector  OutputSignals=SOC (%),Current (A),Voltage (V)
  Product : Product
  Scope : Scope  NumInputPorts=4
      settings: ActiveDisplayYMinimum=99.92989  ActiveDisplayYMaximum=100.00779
  + : PMIOPort  Side=Right
  - : PMIOPort  Port=2  Side=Right
  tag scope: cm_43=global, soc43=global, vm_43=global
  wires:
  Battery1/1 -> Bus Selector/1
  Bus Selector/1 -> [soc43], Scope/1  "<SOC (%)>"
  Product/1 -> Scope/4
  Bus Selector/2 -> [cm_43], Product/1, Scope/2  "<Current (A)>"
  Bus Selector/3 -> [vm_43], Scope/3, Product/2  "<Voltage (V)>"
  connections:
  +/RConn1 -- Battery1/LConn1
  -/RConn1 -- Battery1/LConn2

== system Likitha_Version_3_1/Subsystem11/45 ==
  Battery1 : spsBatteryLib/Battery  BatType=Lithium-Ion  NomV=3.135  NomQ=2.37  SOC=62  Batt_Tr=30  PresetModel=on  MaxQ=2.37  MinV=2.3512  FullV=3.6491  Dis_rate=1.0304  R=0.013228  Normal_OP=2.1433  expZone="[3.387     0.11644]"
  Bus Selector : BusSelector  OutputSignals=SOC (%),Current (A),Voltage (V)
  Product : Product
  Scope : Scope  NumInputPorts=4
      settings: ActiveDisplayYMinimum=99.92989  ActiveDisplayYMaximum=100.00779
  + : PMIOPort  Side=Right
  - : PMIOPort  Port=2  Side=Right
  tag scope: cm_44=global, soc44=global, vm_44=global
  wires:
  Battery1/1 -> Bus Selector/1
  Bus Selector/1 -> [soc44], Scope/1  "<SOC (%)>"
  Product/1 -> Scope/4
  Bus Selector/2 -> [cm_44], Product/1, Scope/2  "<Current (A)>"
  Bus Selector/3 -> [vm_44], Scope/3, Product/2  "<Voltage (V)>"
  connections:
  +/RConn1 -- Battery1/LConn1
  -/RConn1 -- Battery1/LConn2

== system Likitha_Version_3_1/Subsystem11/46 ==
  Battery1 : spsBatteryLib/Battery  BatType=Lithium-Ion  NomV=3.13  NomQ=2.36  SOC=61  Batt_Tr=30  PresetModel=on  MaxQ=2.36  MinV=2.3475  FullV=3.6433  Dis_rate=1.0261  R=0.013263  Normal_OP=2.1343  expZone="[3.3816     0.11595]"
  Bus Selector : BusSelector  OutputSignals=SOC (%),Current (A),Voltage (V)
  Product : Product
  Scope : Scope  NumInputPorts=4
      settings: ActiveDisplayYMinimum=99.92989  ActiveDisplayYMaximum=100.00779
  + : PMIOPort  Side=Right
  - : PMIOPort  Port=2  Side=Right
  tag scope: cm_45=global, soc45=global, vm_45=global
  wires:
  Battery1/1 -> Bus Selector/1
  Bus Selector/1 -> [soc45], Scope/1  "<SOC (%)>"
  Product/1 -> Scope/4
  Bus Selector/2 -> [cm_45], Product/1, Scope/2  "<Current (A)>"
  Bus Selector/3 -> [vm_45], Scope/3, Product/2  "<Voltage (V)>"
  connections:
  +/RConn1 -- Battery1/LConn1
  -/RConn1 -- Battery1/LConn2

== system Likitha_Version_3_1/Subsystem11/47 ==
  Battery1 : spsBatteryLib/Battery  BatType=Lithium-Ion  NomV=3.125  NomQ=2.35  SOC=60  Batt_Tr=30  PresetModel=on  MaxQ=2.35  MinV=2.3438  FullV=3.6375  Dis_rate=1.0217  R=0.013298  Normal_OP=2.1252  expZone="[3.3762     0.11546]"
  Bus Selector : BusSelector  OutputSignals=SOC (%),Current (A),Voltage (V)
  Product : Product
  Scope : Scope  NumInputPorts=4
      settings: ActiveDisplayYMinimum=99.92989  ActiveDisplayYMaximum=100.00779
  + : PMIOPort  Side=Right
  - : PMIOPort  Port=2  Side=Right
  tag scope: cm_46=global, soc46=global, vm_46=global
  wires:
  Battery1/1 -> Bus Selector/1
  Bus Selector/1 -> [soc46], Scope/1  "<SOC (%)>"
  Product/1 -> Scope/4
  Bus Selector/2 -> [cm_46], Product/1, Scope/2  "<Current (A)>"
  Bus Selector/3 -> [vm_46], Scope/3, Product/2  "<Voltage (V)>"
  connections:
  +/RConn1 -- Battery1/LConn1
  -/RConn1 -- Battery1/LConn2

== system Likitha_Version_3_1/Subsystem11/48 ==
  Battery1 : spsBatteryLib/Battery  BatType=Lithium-Ion  NomV=3.12  NomQ=2.34  SOC=59  Batt_Tr=30  PresetModel=on  MaxQ=2.34  MinV=2.34  FullV=3.6316  Dis_rate=1.0174  R=0.013333  Normal_OP=2.1162  expZone="[3.3708     0.11497]"
  Bus Selector : BusSelector  OutputSignals=SOC (%),Current (A),Voltage (V)
  Product : Product
  Scope : Scope  NumInputPorts=4
      settings: ActiveDisplayYMinimum=99.92989  ActiveDisplayYMaximum=100.00779
  + : PMIOPort  Side=Right
  - : PMIOPort  Port=2  Side=Right
  tag scope: cm_47=global, soc47=global, vm_47=global
  wires:
  Battery1/1 -> Bus Selector/1
  Bus Selector/1 -> [soc47], Scope/1  "<SOC (%)>"
  Product/1 -> Scope/4
  Bus Selector/2 -> [cm_47], Product/1, Scope/2  "<Current (A)>"
  Bus Selector/3 -> [vm_47], Scope/3, Product/2  "<Voltage (V)>"
  connections:
  +/RConn1 -- Battery1/LConn1
  -/RConn1 -- Battery1/LConn2

== system Likitha_Version_3_1/Subsystem11/49 ==
  Battery1 : spsBatteryLib/Battery  BatType=Lithium-Ion  NomV=3.115  NomQ=2.33  SOC=58  Batt_Tr=30  PresetModel=on  MaxQ=2.33  MinV=2.3363  FullV=3.6258  Dis_rate=1.013  R=0.013369  Normal_OP=2.1071  expZone="[3.3654     0.11447]"
  Bus Selector : BusSelector  OutputSignals=SOC (%),Current (A),Voltage (V)
  Product : Product
  Scope : Scope  NumInputPorts=4
      settings: ActiveDisplayYMinimum=99.92989  ActiveDisplayYMaximum=100.00779
  + : PMIOPort  Side=Right
  - : PMIOPort  Port=2  Side=Right
  tag scope: cm_48=global, soc48=global, vm_48=global
  wires:
  Battery1/1 -> Bus Selector/1
  Bus Selector/1 -> [soc48], Scope/1  "<SOC (%)>"
  Product/1 -> Scope/4
  Bus Selector/2 -> [cm_48], Product/1, Scope/2  "<Current (A)>"
  Bus Selector/3 -> [vm_48], Scope/3, Product/2  "<Voltage (V)>"
  connections:
  +/RConn1 -- Battery1/LConn1
  -/RConn1 -- Battery1/LConn2

== system Likitha_Version_3_1/Subsystem11/5 ==
  Battery1 : spsBatteryLib/Battery  BatType=Lithium-Ion  NomV=3.3  NomQ=2.7  SOC=98  Batt_Tr=30  PresetModel=on  MaxQ=2.7  MinV=2.475  FullV=3.8412  Dis_rate=1.1739  R=0.012222  Normal_OP=2.4417  expZone="[3.5653     0.13265]"
  Bus Selector : BusSelector  OutputSignals=SOC (%),Current (A),Voltage (V)
  Product : Product
  Scope : Scope  NumInputPorts=4
      settings: ActiveDisplayYMinimum=99.92989  ActiveDisplayYMaximum=100.00779
  + : PMIOPort  Side=Right
  - : PMIOPort  Port=2  Side=Right
  tag scope: cm_5=global, soc5=global, vm_5=global
  wires:
  Battery1/1 -> Bus Selector/1
  Bus Selector/1 -> [soc5], Scope/1  "<SOC (%)>"
  Bus Selector/2 -> Product/1, Scope/2  "<Current (A)>"
  Product/1 -> Scope/4
  Bus Selector/3 -> [vm_5], [cm_5], Scope/3, Product/2  "<Voltage (V)>"
  connections:
  +/RConn1 -- Battery1/LConn1
  -/RConn1 -- Battery1/LConn2

== system Likitha_Version_3_1/Subsystem11/50 ==
  Battery1 : spsBatteryLib/Battery  BatType=Lithium-Ion  NomV=3.11  NomQ=2.32  SOC=57  Batt_Tr=30  PresetModel=on  MaxQ=2.32  MinV=2.3325  FullV=3.62  Dis_rate=1.0087  R=0.013405  Normal_OP=2.0981  expZone="[3.36     0.11398]"
  Bus Selector : BusSelector  OutputSignals=SOC (%),Current (A),Voltage (V)
  Product : Product
  Scope : Scope  NumInputPorts=4
      settings: ActiveDisplayYMinimum=99.92989  ActiveDisplayYMaximum=100.00779
  + : PMIOPort  Side=Right
  - : PMIOPort  Port=2  Side=Right
  tag scope: cm_49=global, soc49=global, vm_49=global
  wires:
  Battery1/1 -> Bus Selector/1
  Bus Selector/1 -> [soc49], Scope/1  "<SOC (%)>"
  Product/1 -> Scope/4
  Bus Selector/2 -> [cm_49], Product/1, Scope/2  "<Current (A)>"
  Bus Selector/3 -> [vm_49], Scope/3, Product/2  "<Voltage (V)>"
  connections:
  +/RConn1 -- Battery1/LConn1
  -/RConn1 -- Battery1/LConn2
